simulink model "PMSM_FOC_F280049C"  (R2024b)
settings: Solver=VariableStepAuto  StartTime=0.0  StopTime=10.0  RelTol=1e-3
PostLoadFcn:
  | parameter_dir = fileparts(get_param(bdroot,'FileName'));
  | run(fullfile(parameter_dir, 'motor_params.m'));
  | run(fullfile(parameter_dir, 'control_params.m'));
  | run(fullfile(parameter_dir, 'simulation_params.m'));
  | MOTOR_VDC = 24.1;
  | clear parameter_dir;
InitFcn:
  | parameter_dir = fileparts(get_param(bdroot,'FileName'));
  | run(fullfile(parameter_dir, 'motor_params.m'));
  | run(fullfile(parameter_dir, 'control_params.m'));
  | run(fullfile(parameter_dir, 'simulation_params.m'));
  | MOTOR_VDC = 24.1;
  | clear parameter_dir;
model workspace (MAT data in the model file):
  MOTOR_VDC = 24.1
undefined symbols (not defined in the file or in its folder): B, flux, J, Ld, Lq, pole_pairs, Rs, Ts
settings Model: Creator=PMSM FOC Public Release  LastModifiedBy=pepsi

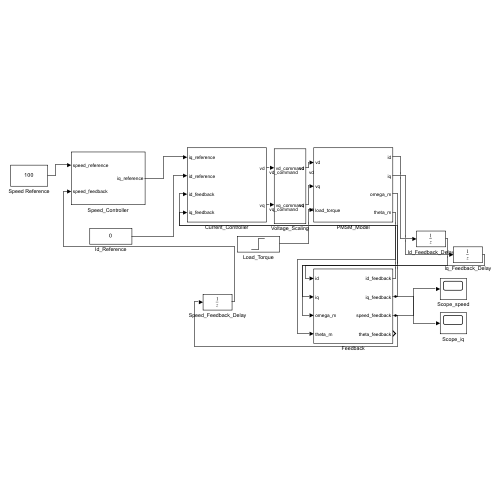
[thumbnail: Simulink's stored preview of the top-level diagram]
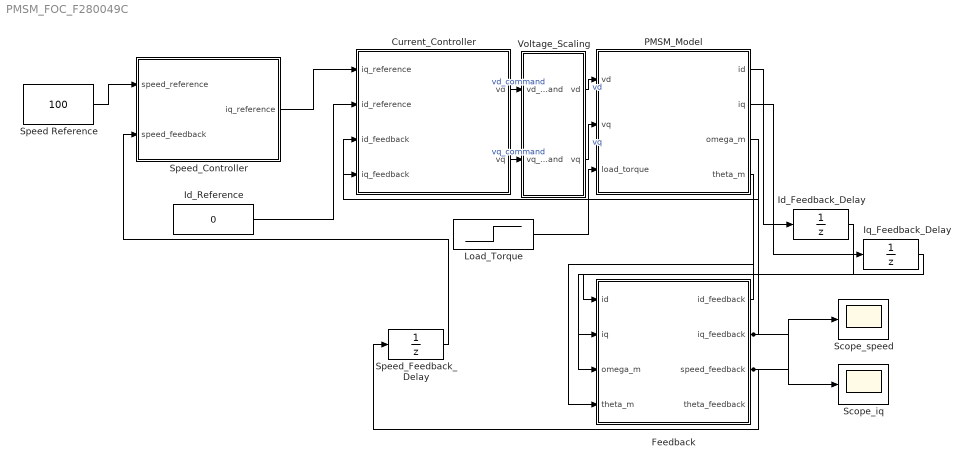
== system PMSM_FOC_F280049C ==
  Current_Controller : Subsystem
  Feedback : Subsystem
  Id_Feedback_Delay : UnitDelay  SampleTime=1/30000  HasFrameUpgradeWarning=on
  Id_Reference : Constant  Value=0
  Iq_Feedback_Delay : UnitDelay  SampleTime=1/30000  HasFrameUpgradeWarning=on
  Load_Torque : Step  Time=3  Before=0.0005  After=0.001  SampleTime=0
  PMSM_Model : Subsystem  InitFcn=parameter_directory = fileparts(get_param(bdroot, 'FileName')); run(fullfile(parameter_directory, 'motor_params.m')); run(fullfile(parameter_directory, 'control_params.m')); run(fullfile(parameter_directory, 'simulation_params.m')); assignin('base', 'Rs', MOTOR_RS_OHM); assignin('base', 'Ld', MOTOR_LD_H); assignin('base', 'Lq', MOTOR_LQ_H); assignin('base', 'flux', MOTOR_FLUX_LINKAGE_WB); assignin('base', 'J', MOTOR_INERTIA_KG_M2); assignin('base', 'B', MOTOR_VISCOUS_FRICTION_NM_S); assignin('base', 'pole_pairs', MOTOR_POLE_PAIRS); assignin('base', 'Ts', 1 / current_loop_frequency);
  Scope_iq : Scope
  Scope_speed : Scope
  Speed Reference : Constant  Value=100
  Speed_Controller : Subsystem
  Speed_Feedback_Delay : UnitDelay  SampleTime=1/30000  HasFrameUpgradeWarning=on
  Voltage_Scaling : Subsystem
  wires:
  Speed_Controller/1(iq_reference) -> Current_Controller/1(iq_reference)
  PMSM_Model/3(omega_m) -> Feedback/3(omega_m)
  PMSM_Model/4(theta_m) -> Feedback/4(theta_m)
  Feedback/1(id_feedback) -> Current_Controller/3(id_feedback)
  Feedback/2(iq_feedback) -> Current_Controller/4(iq_feedback), Scope_iq/1
  Feedback/3(speed_feedback) -> Scope_speed/1, Speed_Feedback_Delay/1
  Id_Reference/1 -> Current_Controller/2(id_reference)
  Current_Controller/1(vd) -> Voltage_Scaling/1(vd_command)  "vd_command"
  Current_Controller/2(vq) -> Voltage_Scaling/2(vq_command)  "vq_command"
  Voltage_Scaling/1(vd) -> PMSM_Model/1(vd)  "vd"
  Voltage_Scaling/2(vq) -> PMSM_Model/2(vq)  "vq"
  PMSM_Model/1(id) -> Id_Feedback_Delay/1
  Id_Feedback_Delay/1 -> Feedback/1(id)
  PMSM_Model/2(iq) -> Iq_Feedback_Delay/1
  Iq_Feedback_Delay/1 -> Feedback/2(iq)
  Speed_Feedback_Delay/1 -> Speed_Controller/2(speed_feedback)
  Load_Torque/1 -> PMSM_Model/3(load_torque)
  Speed Reference/1 -> Speed_Controller/1(speed_reference)

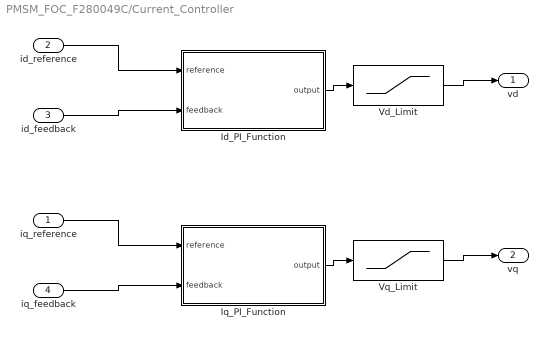
== system PMSM_FOC_F280049C/Current_Controller ==
  iq_reference : Inport
  id_reference : Inport  Port=2
  id_feedback : Inport  Port=3
  iq_feedback : Inport  Port=4
  Id_PI_Function : MATLAB Function  TreatAsAtomicUnit=on
  Iq_PI_Function : MATLAB Function  TreatAsAtomicUnit=on
  Vd_Limit : Saturate  UpperLimit=0.010  LowerLimit=-0.010
  Vq_Limit : Saturate  UpperLimit=0.100  LowerLimit=-0.100
  vd : Outport
  vq : Outport  Port=2
  wires:
  id_reference/1 -> Id_PI_Function/1(reference)
  id_feedback/1 -> Id_PI_Function/2(feedback)
  Id_PI_Function/1(output) -> Vd_Limit/1
  Vd_Limit/1 -> vd/1
  iq_reference/1 -> Iq_PI_Function/1(reference)
  iq_feedback/1 -> Iq_PI_Function/2(feedback)
  Iq_PI_Function/1(output) -> Vq_Limit/1
  Vq_Limit/1 -> vq/1

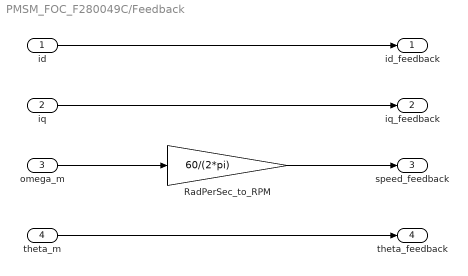
== system PMSM_FOC_F280049C/Feedback ==
  id : Inport
  iq : Inport  Port=2
  omega_m : Inport  Port=3
  theta_m : Inport  Port=4
  RadPerSec_to_RPM : Gain  Gain=60/(2*pi)
  id_feedback : Outport
  iq_feedback : Outport  Port=2
  speed_feedback : Outport  Port=3
  theta_feedback : Outport  Port=4
  wires:
  id/1 -> id_feedback/1
  iq/1 -> iq_feedback/1
  omega_m/1 -> RadPerSec_to_RPM/1
  RadPerSec_to_RPM/1 -> speed_feedback/1
  theta_m/1 -> theta_feedback/1

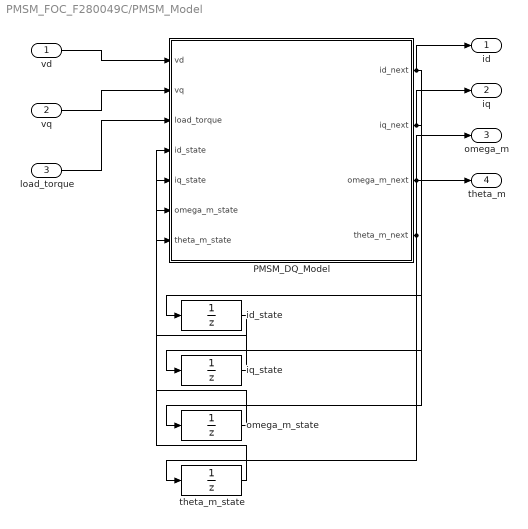
== system PMSM_FOC_F280049C/PMSM_Model ==
  vd : Inport
  vq : Inport  Port=2
  load_torque : Inport  Port=3
  PMSM_DQ_Model : MATLAB Function  TreatAsAtomicUnit=on
  id_state : UnitDelay  SampleTime=-1  HasFrameUpgradeWarning=on
  iq_state : UnitDelay  SampleTime=-1  HasFrameUpgradeWarning=on
  omega_m_state : UnitDelay  SampleTime=-1  HasFrameUpgradeWarning=on
  theta_m_state : UnitDelay  SampleTime=-1  HasFrameUpgradeWarning=on
  id : Outport
  iq : Outport  Port=2
  omega_m : Outport  Port=3
  theta_m : Outport  Port=4
  wires:
  vd/1 -> PMSM_DQ_Model/1(vd)
  vq/1 -> PMSM_DQ_Model/2(vq)
  load_torque/1 -> PMSM_DQ_Model/3(load_torque)
  PMSM_DQ_Model/1(id_next) -> id/1, id_state/1
  PMSM_DQ_Model/2(iq_next) -> iq/1, iq_state/1
  PMSM_DQ_Model/3(omega_m_next) -> omega_m/1, omega_m_state/1
  PMSM_DQ_Model/4(theta_m_next) -> theta_m/1, theta_m_state/1
  id_state/1 -> PMSM_DQ_Model/4(id_state)
  iq_state/1 -> PMSM_DQ_Model/5(iq_state)
  omega_m_state/1 -> PMSM_DQ_Model/6(omega_m_state)
  theta_m_state/1 -> PMSM_DQ_Model/7(theta_m_state)

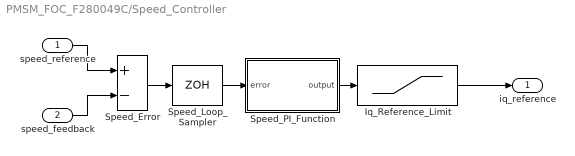
== system PMSM_FOC_F280049C/Speed_Controller ==
  speed_reference : Inport
  speed_feedback : Inport  Port=2
  Iq_Reference_Limit : Saturate  UpperLimit=0.120  LowerLimit=-0.120
  Speed_Error : Sum  Inputs=+-
  Speed_Loop_Sampler : ZeroOrderHold  SampleTime=0.01
  Speed_PI_Function : MATLAB Function  TreatAsAtomicUnit=on
  iq_reference : Outport
  wires:
  speed_reference/1 -> Speed_Error/1
  speed_feedback/1 -> Speed_Error/2
  Iq_Reference_Limit/1 -> iq_reference/1
  Speed_Error/1 -> Speed_Loop_Sampler/1
  Speed_Loop_Sampler/1 -> Speed_PI_Function/1(error)
  Speed_PI_Function/1(output) -> Iq_Reference_Limit/1

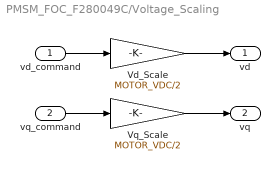
== system PMSM_FOC_F280049C/Voltage_Scaling ==
  vd_command : Inport
  vq_command : Inport  Port=2
  Vd_Scale : Gain  Gain=MOTOR_VDC/2
  Vq_Scale : Gain  Gain=MOTOR_VDC/2
  vd : Outport
  vq : Outport  Port=2
  wires:
  vd_command/1 -> Vd_Scale/1
  Vd_Scale/1 -> vd/1
  vq_command/1 -> Vq_Scale/1
  Vq_Scale/1 -> vq/1

== matlab function PMSM_FOC_F280049C/Current_Controller/Id_PI_Function ==
  data: reference input; output output; feedback input
function output = fcn(reference, feedback)
%#codegen
persistent integrator
if isempty(integrator)
    integrator = 0.0;
end
Kp = 0.15;
Ki = 0.00050;
limit = 0.010;
error = reference - feedback;
p_term = Kp * error;
integrator_candidate = integrator + Ki * error;
unsat_output = p_term + integrator_candidate;
sat_output = unsat_output;
if sat_output > limit
    sat_output = limit;
elseif sat_output < -limit
    sat_output = -limit;
end
if (unsat_output == sat_output) || ...
        ((unsat_output > limit) && (error < 0.0)) || ...
        ((unsat_output < -limit) && (error > 0.0))
    integrator = integrator_candidate;
end
output = p_term + integrator;
if output > limit
    output = limit;
elseif output < -limit
    output = -limit;
end
end

== matlab function PMSM_FOC_F280049C/PMSM_Model/PMSM_DQ_Model ==
  data: vd input double size=1; id_next output; vq input double size=1; load_torque input double size=1; id_state input double size=1; iq_state input double size=1; omega_m_state input double size=1; theta_m_state input double size=1; iq_next output; omega_m_next output; theta_m_next output; Rs parameter; Ld parameter; Lq parameter; flux parameter; J parameter; B parameter; pole_pairs parameter; Ts parameter
function [id_next, iq_next, omega_m_next, theta_m_next] = fcn(vd, vq, load_torque, id_state, iq_state, omega_m_state, theta_m_state, Rs, Ld, Lq, flux, J, B, pole_pairs, Ts)
%#codegen
omega_e = pole_pairs * omega_m_state;
did_dt = (vd - Rs * id_state + omega_e * Lq * iq_state) / Ld;
diq_dt = (vq - Rs * iq_state - omega_e * (Ld * id_state + flux)) / Lq;
Te = 1.5 * pole_pairs * (flux * iq_state + (Ld - Lq) * id_state * iq_state);
domega_m_dt = (Te - load_torque - B * omega_m_state) / J;
id_next = double(id_state + did_dt * Ts);
iq_next = double(iq_state + diq_dt * Ts);
omega_m_next = double(omega_m_state + domega_m_dt * Ts);
theta_m_next = double(theta_m_state + omega_m_next * Ts);
end

== matlab function PMSM_FOC_F280049C/Current_Controller/Iq_PI_Function ==
  data: reference input; output output; feedback input
function output = fcn(reference, feedback)
%#codegen
persistent integrator
if isempty(integrator)
    integrator = 0.0;
end
Kp = 0.15;
Ki = 0.00050;
limit = 0.100;
error = reference - feedback;
p_term = Kp * error;
integrator_candidate = integrator + Ki * error;
unsat_output = p_term + integrator_candidate;
sat_output = unsat_output;
if sat_output > limit
    sat_output = limit;
elseif sat_output < -limit
    sat_output = -limit;
end
if (unsat_output == sat_output) || ...
        ((unsat_output > limit) && (error < 0.0)) || ...
        ((unsat_output < -limit) && (error > 0.0))
    integrator = integrator_candidate;
end
output = p_term + integrator;
if output > limit
    output = limit;
elseif output < -limit
    output = -limit;
end
end

== matlab function PMSM_FOC_F280049C/Speed_Controller/Speed_PI_Function ==
  data: error input; output output
function output = fcn(error)
%#codegen
persistent integrator
if isempty(integrator)
    integrator = 0.0;
end
Kp = 0.00040;
Ki = 0.000010;
limit = 0.120;
p_term = Kp * error;
integrator_candidate = integrator + Ki * error;
unsat_output = p_term + integrator_candidate;
sat_output = unsat_output;
if sat_output > limit
    sat_output = limit;
elseif sat_output < -limit
    sat_output = -limit;
end
if (unsat_output == sat_output) || ...
        ((unsat_output > limit) && (error < 0.0)) || ...
        ((unsat_output < -limit) && (error > 0.0))
    integrator = integrator_candidate;
end
output = p_term + integrator;
if output > limit
    output = limit;
elseif output < -limit
    output = -limit;
end
end
